simulink model "impedance_new"  (Simulink 8.5)
settings: Solver=ode15s  SolverMode=SingleTasking  StartTime=0.0  StopTime=0.1  RelTol=1e-3  AbsTol=1e-6
libraries: powerlib x25
settings Model: Creator=PC  LastModifiedBy=PC  ExtModeTrigMode=oneshot  ExtModeArmWhenConnect=off
settings DataIOCC: LimitDataPoints=off
settings OptimizationCC: BlockReduction=off  BooleanDataType=off  ExpressionDepthLimit=128
settings DebuggingCC: SaveWithParameterizedLinksMsg=none  SignalResolutionControl=TryResolveAllWithWarning  MultiTaskDSMMsg=warning  MultiTaskCondExecSysMsg=none  FcnCallInpInsideContextMsg=EnableAllAsError  UnconnectedLineMsg=none  StateNameClashWarn=none
settings HardwareCC: TargetUnknown=on

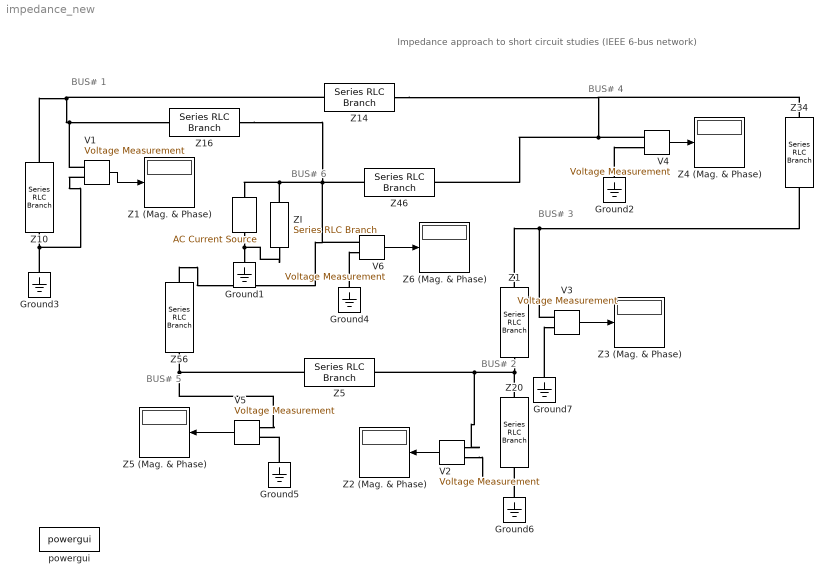
== system impedance_new ==
  note: Impedance approach to short circuit studies
      | (IEEE 6-bus network)
  note: BUS# 4
  note: BUS# 1
  note: BUS# 6
  note: BUS# 5
  note: BUS# 2
  note: BUS# 3
  " " : powerlib/Electrical Sources/AC Current Source  Amplitude=1  Phase=0  Frequency=60  SampleTime=0  Measurements=None
  Ground{1..7} (7 alike) : powerlib/Elements/Ground  LConnTagsString=a
  V{1..6} (6 alike) : powerlib/Measurements/Voltage Measurement  PhasorSimulation=off  OutputType=Complex  PSBequivalent=0
  Z1 : powerlib/Elements/Series RLC Branch  LConnTagsString=__new0  RConnTagsString=__new0  BranchType=RL  Resistance=1.446  Inductance=2.1/(2*pi*60)  SetiL0=off  InitialCurrent=0  Capacitance=1e-6  Setx0=off  InitialVoltage=0  Measurements=None
  Z1 (Mag. & Phase) : Display
  Z10 : powerlib/Elements/Series RLC Branch  LConnTagsString=__new0  RConnTagsString=__new0  BranchType=RL  Resistance=0.02  Inductance=0.24/(2*pi*60)  SetiL0=off  InitialCurrent=0  Capacitance=1e-6  Setx0=off  InitialVoltage=0  Measurements=None
  Z14 : powerlib/Elements/Series RLC Branch  LConnTagsString=__new0  RConnTagsString=__new0  BranchType=RL  Resistance=0.16  Inductance=0.74/(2*pi*60)  SetiL0=off  InitialCurrent=0  Capacitance=1e-6  Setx0=off  InitialVoltage=0  Measurements=None
  Z16 : powerlib/Elements/Series RLC Branch  LConnTagsString=__new0  RConnTagsString=__new0  BranchType=RL  Resistance=0.246  Inductance=1.036/(2*pi*60)  SetiL0=off  InitialCurrent=0  Capacitance=1e-6  Setx0=off  InitialVoltage=0  Measurements=None
  Z2 (Mag. & Phase) : Display
  Z20 : powerlib/Elements/Series RLC Branch  LConnTagsString=__new0  RConnTagsString=__new0  BranchType=RL  Resistance=0.03  Inductance=0.48/(2*pi*60)  SetiL0=off  InitialCurrent=0  Capacitance=1e-6  Setx0=off  InitialVoltage=0  Measurements=None
  Z3 (Mag. & Phase) : Display
  Z34 : powerlib/Elements/Series RLC Branch  LConnTagsString=__new0  RConnTagsString=__new0  BranchType=RL  Resistance=0  Inductance=0.266/(2*pi*60)  SetiL0=off  InitialCurrent=0  Capacitance=1e-6  Setx0=off  InitialVoltage=0  Measurements=None
  Z4 (Mag. & Phase) : Display
  Z46 : powerlib/Elements/Series RLC Branch  LConnTagsString=__new0  RConnTagsString=__new0  BranchType=RL  Resistance=0.194  Inductance=0.814/(2*pi*60)  SetiL0=off  InitialCurrent=0  Capacitance=1e-6  Setx0=off  InitialVoltage=0  Measurements=None
  Z5 : powerlib/Elements/Series RLC Branch  LConnTagsString=__new0  RConnTagsString=__new0  BranchType=RL  Resistance=0.564  Inductance=1.28/(2*pi*60)  SetiL0=off  InitialCurrent=0  Capacitance=1e-6  Setx0=off  InitialVoltage=0  Measurements=None
  Z5 (Mag. & Phase) : Display
  Z56 : powerlib/Elements/Series RLC Branch  LConnTagsString=__new0  RConnTagsString=__new0  BranchType=RL  Resistance=0  Inductance=0.6/(2*pi*60)  SetiL0=off  InitialCurrent=0  Capacitance=1e-6  Setx0=off  InitialVoltage=0  Measurements=None
  Z6 (Mag. & Phase) : Display
  ZI : powerlib/Elements/Series RLC Branch  LConnTagsString=__new0  RConnTagsString=__new0  BranchType=R  Resistance=1000000  Inductance=0.48/(2*pi*60)  SetiL0=off  InitialCurrent=0  Capacitance=1e-6  Setx0=off  InitialVoltage=0  Measurements=None
  powergui : powerlib/powergui  SimulationMode=Continuous  SolverType=Tustin/Backward Euler (TBE)  SampleTime=0  frequency=60  SPID=off  DisableSnubberDevices=off  DisableRonSwitches=off  DisableVfSwitches=off  SwTol=0  DisplayEquations=off  Interpol=off  methode=off  Ts=0  FunctionMessages=off  echomessages=off  HookPort=off  EnableUseOfTLC=off  x0status=blocks  frequencyindice=60  Pbase=100e6  ErrMax=1e-4  Iterations=50  UnitsV=kV  UnitsW=MW  buscounter=0  RestoreLinks=warning  ResistiveCurrentMeasurement=off  Frange=[0:2:500]  Ylog=off  Xlog=on  ShowGrid=off  save=off  variable=ZData  structure=0  ZoomFFT=on  StartTime=0.0  cycles=1  DisplayStyle=1  fundamental=60  FreqAxis=off  MaxFrequency=1000  frequencyindicesteady=1  RmsSteady=1  display=off
  wires:
  V1/1 -> Z1 (Mag. & Phase)/1
  V2/1 -> Z2 (Mag. & Phase)/1
  V3/1 -> Z3 (Mag. & Phase)/1
  V5/1 -> Z5 (Mag. & Phase)/1
  V6/1 -> Z6 (Mag. & Phase)/1
  V4/1 -> Z4 (Mag. & Phase)/1
  connections:
  " "/LConn1 -- ZI/RConn1 -- Ground1/LConn1
  Z46/LConn1 -- V6/LConn1 -- Z56/LConn1 -- Z16/LConn1 -- ZI/LConn1 -- " "/RConn1
  Ground2/LConn1 -- V4/LConn2
  V4/LConn1 -- Z14/RConn1 -- Z34/LConn1 -- Z46/RConn1
  Z14/LConn1 -- Z10/LConn1 -- V1/LConn1 -- Z16/RConn1
  Ground3/LConn1 -- V1/LConn2 -- Z10/RConn1
  Ground4/LConn1 -- V6/LConn2
  Ground5/LConn1 -- V5/LConn2
  V5/LConn1 -- Z56/RConn1 -- Z5/LConn1
  Z1/RConn1 -- Z20/LConn1 -- V2/LConn1 -- Z5/RConn1
  Ground6/LConn1 -- V2/LConn2 -- Z20/RConn1
  Ground7/LConn1 -- V3/LConn2
  Z1/LConn1 -- V3/LConn1 -- Z34/RConn1
